simulink model "house_model1"  (Simulink 7.6)
settings: Solver=ode45  StartTime=0.0  StopTime=4*3600  RelTol=1e-3
values from neighbouring files (symbols this model uses):
  C_R = 100000    [Simulation.m]
  K = 100    [Simulation.m]
  Q_F_ON = 1000    [Simulation.m]
  Q_H = 1500    [Simulation.m]
  t_a = 0    [Simulation.m]
  t_init = 5    [Simulation.m]
  tau_F = 2*3600    (= 7200)    [Simulation.m]
settings Model: Creator=sgt  LastModifiedBy=sgt
settings OptimizationCC: InlineInvariantSignals=on  InitFltsAndDblsToZero=on
settings DebuggingCC: SaveWithParameterizedLinksMsg=none  SignalResolutionControl=TryResolveAllWithWarning  MultiTaskDSMMsg=warning  MultiTaskCondExecSysMsg=none  StrictBusMsg=None
settings RTWCC: IncludeERTFirstTime=on
settings GRTTargetCC: TargetFcnLib=ansi_tfl_tmw.mat

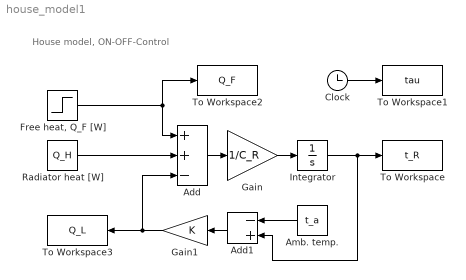
== system house_model1 ==
  note: House model, ON-OFF-Control
  Add : Sum  Inputs=++-
  Add1 : Sum  Inputs=-+
  Amb. temp. : Constant  Value=t_a
  Clock : Clock
      settings: Decimation=10
  "Free heat, Q_F [W]" : Step  Time=tau_F  After=Q_F_ON  SampleTime=0
  Gain : Gain  Gain=1/C_R
  Gain1 : Gain  Gain=K
  Integrator : Integrator  InitialCondition=t_init
  Radiator heat [W] : Constant  Value=Q_H
  To Workspace : ToWorkspace  VariableName=t_R  SampleTime=-1  SaveFormat=Array
  To Workspace1 : ToWorkspace  VariableName=tau  SampleTime=-1  SaveFormat=Array
  To Workspace2 : ToWorkspace  VariableName=Q_F  SampleTime=-1  SaveFormat=Array
  To Workspace3 : ToWorkspace  VariableName=Q_L  SampleTime=-1  SaveFormat=Array
  wires:
  Integrator/1 -> Add1/2, To Workspace/1
  Clock/1 -> To Workspace1/1
  Gain/1 -> Integrator/1
  Add/1 -> Gain/1
  "Free heat, Q_F [W]"/1 -> Add/1, To Workspace2/1
  Amb. temp./1 -> Add1/1
  Add1/1 -> Gain1/1
  Gain1/1 -> Add/3, To Workspace3/1
  Radiator heat [W]/1 -> Add/2
